simulink model "ClosedLoopStim_SimulatedInput_WithDecoderModel"  (R2016b)
settings: Solver=FixedStepDiscrete  StartTime=0.0  StopTime=inf  FixedStep=sCoreParams.core.stepPeriod  RelTol=1e-3  EnableMultiTasking=on
undefined symbols (not defined in the file or in its folder): sCoreParams, sCoreParams_Features_Baseline_thresholdAboveValue, sCoreParams_Features_Baseline_thresholdBelowValue
libraries: dspswit3 x4, dspsrcs4 x2, simulink x1
settings Model: DataTypeOverride=Double  MinMaxOverflowLogging=ForceOff  Creator=rzelmann  LastModifiedBy=rzelmann
settings SolverCC: EnableConcurrentExecution=on  ConcurrentTasks=on  AutoInsertRateTranBlk=on  InsertRTBMode=Always
settings DataIOCC: SaveFormat=StructureWithTime  SaveOutput=off  SignalLogging=off  DSMLogging=off  SaveTime=off
settings OptimizationCC: BlockReduction=off  OptimizeBlockIOStorage=off  BufferReuse=off  GlobalBufferReuse=off  ExpressionFolding=off  LocalBlockOutputs=off  LifeSpan=inf
settings DebuggingCC: AllowSymbolicDim=off  SFUnexpectedBacktrackingDiag=warning  SFNoUnconditionalDefaultTransitionDiag=warning  SFExecutionAtInitializationDiag=none
settings HardwareCC: ProdBitPerPointer=32  ProdBitPerSizeT=32  ProdBitPerPtrDiffT=32  ProdLargestAtomicFloat=None  ProdWordSize=32  ProdLongLongMode=on  ProdHWDeviceType=Generic->32-bit x86 compatible
settings RTWCC: SystemTargetFile=slrt.tlc  TemplateMakefile=slrt_default_tmf  Description=Simulink Real-Time  RTWCompilerOptimization=on
settings CodeAppCC: MaxIdLength=63
settings ConfigComp: CovMetricSettings=dw  CovHtmlReporting=on  CovSaveCumulativeToWorkspaceVar=on  CovSaveSingleToWorkspaceVar=on  CovExternalEMLEnable=off

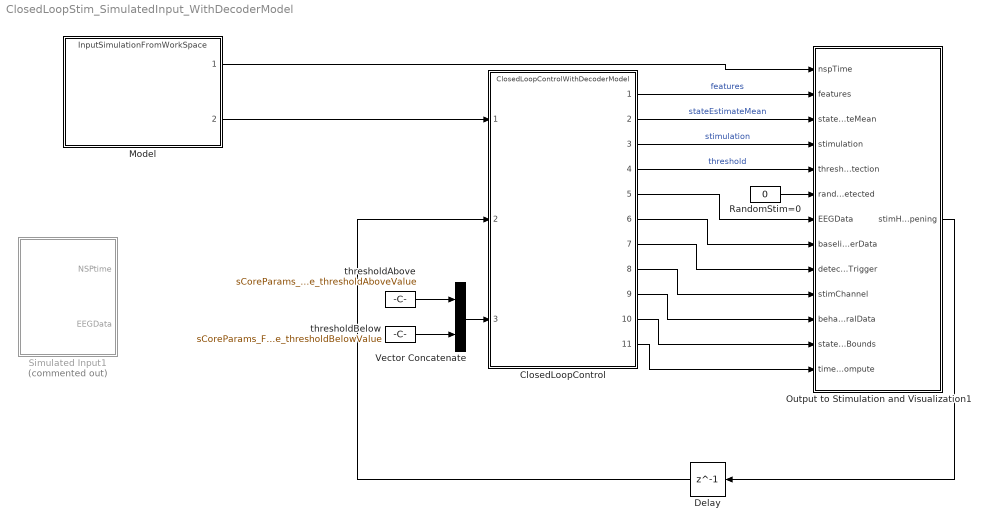
== system ClosedLoopStim_SimulatedInput_WithDecoderModel ==
  ClosedLoopControl : ModelReference  ModelNameDialog=ClosedLoopControlWithDecoderModel.slx  SimulationMode=Normal  ModelReferenceVersion=1.730
  Delay : Delay  DelayLength=1  InitialCondition=0  InputProcessing=Columns as channels (frame based)  SampleTime=sCoreParams.core.stepPeriod
  Model : ModelReference  ModelNameDialog=InputSimulationFromWorkSpace.slx  SimulationMode=Normal  ModelReferenceVersion=1.12
  Output to Stimulation and Visualization1 : Subsystem
  RandomStim=0 : Constant  Value=0  OutDataTypeStr=boolean
  Simulated Input1 : Subsystem  Commented=on
  Vector Concatenate : Concatenate
  thresholdAbove : Constant  Value=sCoreParams_Features_Baseline_thresholdAboveValue
  thresholdBelow : Constant  Value=sCoreParams_Features_Baseline_thresholdBelowValue
  wires:
  Delay/1 -> ClosedLoopControl/2
  ClosedLoopControl/8 -> Output to Stimulation and Visualization1/10(stimChannel)
  ClosedLoopControl/1 -> Output to Stimulation and Visualization1/2(features)  "features"
  ClosedLoopControl/2 -> Output to Stimulation and Visualization1/3(stateEstimateMean)  "stateEstimateMean"
  ClosedLoopControl/3 -> Output to Stimulation and Visualization1/4(stimulation)  "stimulation"
  ClosedLoopControl/4 -> Output to Stimulation and Visualization1/5(thresholdUsedInDetection)  "threshold"
  ClosedLoopControl/6 -> Output to Stimulation and Visualization1/8(baselineTriggerData)
  ClosedLoopControl/7 -> Output to Stimulation and Visualization1/9(detectStimTrigger)
  RandomStim=0/1 -> Output to Stimulation and Visualization1/6(randomDetected)
  ClosedLoopControl/5 -> Output to Stimulation and Visualization1/7(EEGData)
  thresholdAbove/1 -> Vector Concatenate/1
  thresholdBelow/1 -> Vector Concatenate/2
  Vector Concatenate/1 -> ClosedLoopControl/3
  ClosedLoopControl/10 -> Output to Stimulation and Visualization1/12(stateEstimateBounds)
  Output to Stimulation and Visualization1/1(stimHappening) -> Delay/1
  ClosedLoopControl/9 -> Output to Stimulation and Visualization1/11(behavioralData)
  ClosedLoopControl/11 -> Output to Stimulation and Visualization1/13(timeToCompute)
  Model/1 -> Output to Stimulation and Visualization1/1(nspTime)
  Model/2 -> ClosedLoopControl/1

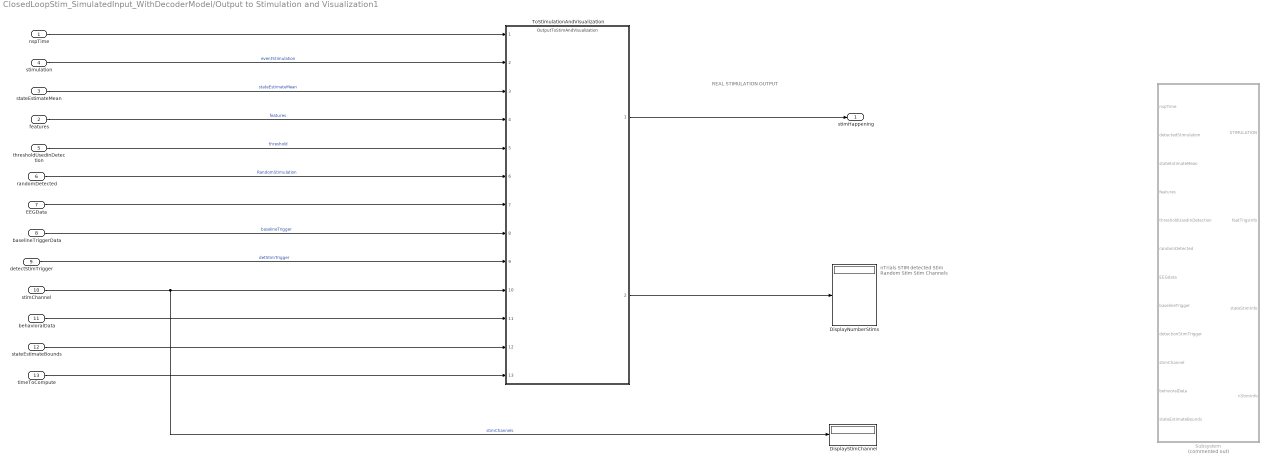
== system ClosedLoopStim_SimulatedInput_WithDecoderModel/Output to Stimulation and Visualization1 ==
  note: nTrials
      | STIM
      | detected Stim
      | Random Stim
      | Stim Channels
  note: REAL STIMULATION OUTPUT
  nspTime : Inport
  features : Inport  Port=2
  stateEstimateMean : Inport  Port=3
  stimulation : Inport  Port=4
  thresholdUsedInDetection : Inport  Port=5
  randomDetected : Inport  Port=6
  EEGData : Inport  Port=7
  baselineTriggerData : Inport  Port=8  OutDataTypeStr=int32
  detectStimTrigger : Inport  Port=9  OutDataTypeStr=int32
  stimChannel : Inport  Port=10
  behavioralData : Inport  Port=11
  stateEstimateBounds : Inport  Port=12
  timeToCompute : Inport  Port=13  OutDataTypeStr=boolean
  DisplayNumberStims : Display
      settings: Format=decimal (Stored Integer)
  DisplayStimChannel : Display
  Subsystem : Subsystem  Commented=on
  ToStimulationAndVisualization : ModelReference  ModelNameDialog=OutputToStimAndVisualization.slx  SimulationMode=Normal  ModelReferenceVersion=1.301
  stimHappening : Outport  OutDataTypeStr=boolean  SampleTime=sCoreParams.core.stepPeriod
  wires:
  stimChannel/1 -> ToStimulationAndVisualization/10, DisplayStimChannel/1  "stimChannels"
  ToStimulationAndVisualization/2 -> DisplayNumberStims/1
  nspTime/1 -> ToStimulationAndVisualization/1
  stimulation/1 -> ToStimulationAndVisualization/2  "eventStimulation"
  stateEstimateMean/1 -> ToStimulationAndVisualization/3  "stateEstimateMean"
  features/1 -> ToStimulationAndVisualization/4  "features"
  thresholdUsedInDetection/1 -> ToStimulationAndVisualization/5  "threshold"
  randomDetected/1 -> ToStimulationAndVisualization/6  "RandomStimulation"
  EEGData/1 -> ToStimulationAndVisualization/7
  baselineTriggerData/1 -> ToStimulationAndVisualization/8  "baselineTrigger"
  detectStimTrigger/1 -> ToStimulationAndVisualization/9  "detStimTrigger"
  behavioralData/1 -> ToStimulationAndVisualization/11
  stateEstimateBounds/1 -> ToStimulationAndVisualization/12
  ToStimulationAndVisualization/1 -> stimHappening/1
  timeToCompute/1 -> ToStimulationAndVisualization/13

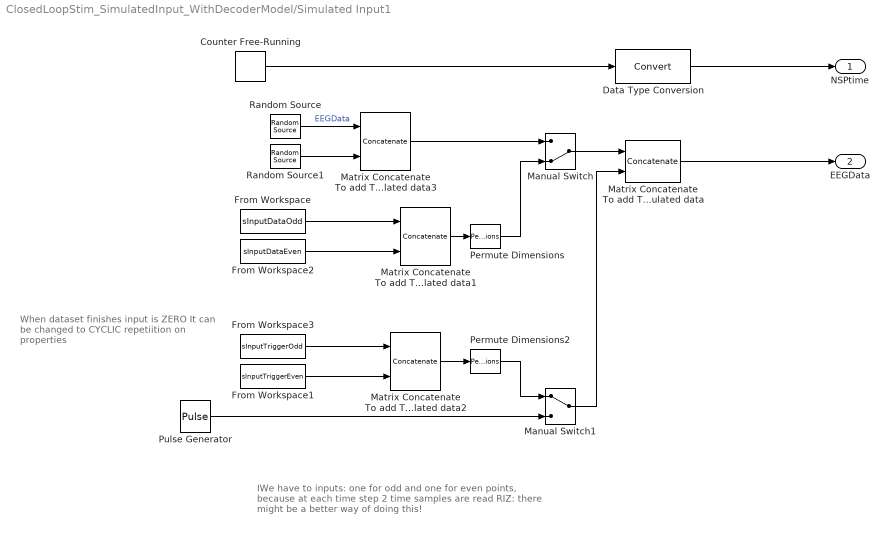
== system ClosedLoopStim_SimulatedInput_WithDecoderModel/Simulated Input1 ==
  note: When dataset finishes input is ZERO
      | It can be changed to CYCLIC repetiition
      | on properties
  note: IWe have to inputs:
      | one for odd and one for even points, because at each time step 2 time samples are read
      | RIZ: there might be a better way of doing this!
  Counter Free-Running : simulink/Sources/Counter Free-Running  NumBits=64  tsamp=sCoreParams.core.stepPeriod
  Data Type Conversion : DataTypeConversion
  From Workspace : FromWorkspace  VariableName=sInputDataOdd  SampleTime=sCoreParams.core.stepPeriod  Interpolate=off  OutputAfterFinalValue=Setting to zero
  From Workspace1 : FromWorkspace  VariableName=sInputTriggerEven  SampleTime=sCoreParams.core.stepPeriod  Interpolate=off  OutputAfterFinalValue=Setting to zero
  From Workspace2 : FromWorkspace  VariableName=sInputDataEven  SampleTime=sCoreParams.core.stepPeriod  Interpolate=off  OutputAfterFinalValue=Setting to zero
  From Workspace3 : FromWorkspace  VariableName=sInputTriggerOdd  SampleTime=sCoreParams.core.stepPeriod  Interpolate=off  OutputAfterFinalValue=Setting to zero
  Manual Switch : ManualSwitch  CurrentSetting=0
  Manual Switch1 : ManualSwitch
  Matrix Concatenate To add Trigger after simulated data : Concatenate  Mode=Multidimensional array  ConcatenateDimension=2
  Matrix Concatenate To add Trigger after simulated data1 : Concatenate  Mode=Multidimensional array  ConcatenateDimension=2
  Matrix Concatenate To add Trigger after simulated data2 : Concatenate  Mode=Multidimensional array  ConcatenateDimension=2
  Matrix Concatenate To add Trigger after simulated data3 : Concatenate  Mode=Multidimensional array
  Permute Dimensions : PermuteDimensions
  Permute Dimensions2 : PermuteDimensions
  Pulse Generator : DiscretePulseGenerator  Amplitude=ones(2,2)  Period=sCoreParams.core.samplingRate * 10  SampleTime=sCoreParams.core.stepPeriod  VectorParams1D=off
  Random Source : dspsrcs4/Random Source  SrcType=Uniform  NormMethod=Ziggurat  CltLength=12  MinVal=-10 * ones(1, sCoreParams.core.maxChannelsAllNSPs-2)  MaxVal=10 * ones(1, sCoreParams.core.maxChannelsAllNSPs-2)  MeanVal=0  VarVal=1  RepMode=Not repeatable  rawSeed=1  IsInherit=off  SampMode=Discrete  SampTime=sCoreParams.core.stepPeriod  SampFrame=1  DataType=Double  OutComplex=Real  OutputFrames=off
  Random Source1 : dspsrcs4/Random Source  SrcType=Uniform  NormMethod=Ziggurat  CltLength=12  MinVal=-10 * ones(1, sCoreParams.core.maxChannelsAllNSPs-2)  MaxVal=10 * ones(1, sCoreParams.core.maxChannelsAllNSPs-2)  MeanVal=0  VarVal=1  RepMode=Not repeatable  rawSeed=1  IsInherit=off  SampMode=Discrete  SampTime=sCoreParams.core.stepPeriod  SampFrame=1  DataType=Double  OutComplex=Real  OutputFrames=off
  NSPtime : Outport
  EEGData : Outport  Port=2
  wires:
  Manual Switch/1 -> Matrix Concatenate To add Trigger after simulated data/1
  Manual Switch1/1 -> Matrix Concatenate To add Trigger after simulated data/2
  Counter Free-Running/1 -> Data Type Conversion/1
  Random Source/1 -> Matrix Concatenate To add Trigger after simulated data3/1  "EEGData"
  Data Type Conversion/1 -> NSPtime/1
  Pulse Generator/1 -> Manual Switch1/2
  Matrix Concatenate To add Trigger after simulated data/1 -> EEGData/1
  Matrix Concatenate To add Trigger after simulated data2/1 -> Permute Dimensions2/1
  From Workspace/1 -> Matrix Concatenate To add Trigger after simulated data1/1
  From Workspace3/1 -> Matrix Concatenate To add Trigger after simulated data2/1
  Matrix Concatenate To add Trigger after simulated data1/1 -> Permute Dimensions/1
  Permute Dimensions/1 -> Manual Switch/2
  Random Source1/1 -> Matrix Concatenate To add Trigger after simulated data3/2
  Matrix Concatenate To add Trigger after simulated data3/1 -> Manual Switch/1
  Permute Dimensions2/1 -> Manual Switch1/1
  From Workspace2/1 -> Matrix Concatenate To add Trigger after simulated data1/2
  From Workspace1/1 -> Matrix Concatenate To add Trigger after simulated data2/2

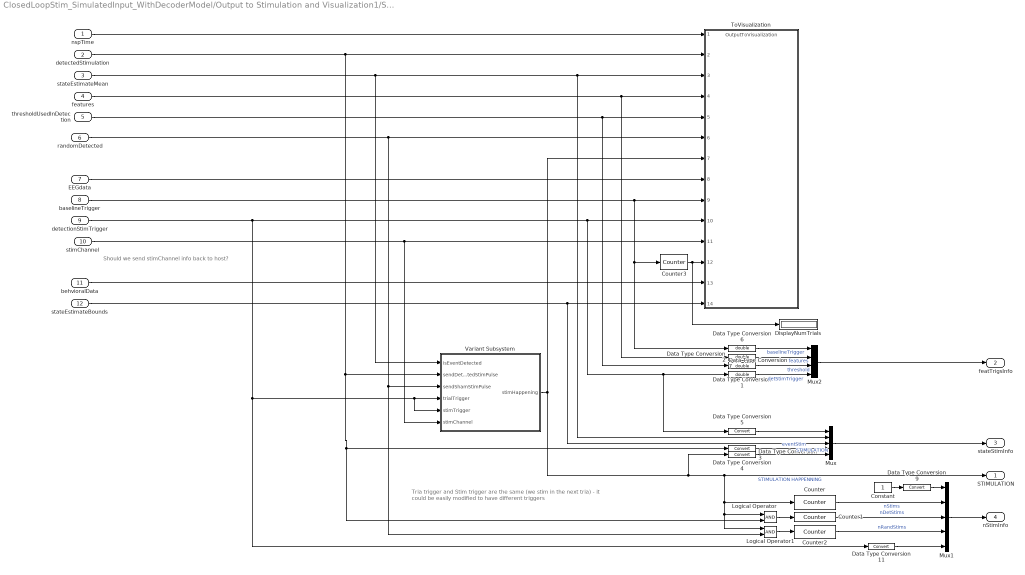
== system ClosedLoopStim_SimulatedInput_WithDecoderModel/Output to Stimulation and Visualization1/Subsystem ==
  note: Should we send stimChannel info back to host?
  note: Tria trigger and Stim trigger are the same (we stim in the next tria)
      | - it could be easily modified to have different triggers
  nspTime : Inport
  detectedStimulation : Inport  Port=2
  stateEstimateMean : Inport  Port=3
  features : Inport  Port=4
  thresholdUsedInDetection : Inport  Port=5
  randomDetected : Inport  Port=6
  EEGdata : Inport  Port=7
  baselineTrigger : Inport  Port=8
  detectionStimTrigger : Inport  Port=9
  stimChannel : Inport  Port=10
  behvioralData : Inport  Port=11
  stateEstimateBounds : Inport  Port=12
  Constant : Constant  OutDataTypeStr=int32
  Counter : dspswit3/Counter  Direction=Up  CountEvent=Rising edge  CounterSize=User defined  MaxCount=1024  InitialCount=0  Output=Count  HitValue=32  ResetInput=off  SamplesPerFrame=1  Ts=1  CntDtype=int32  HitDtype=Logical
  Counter1 : dspswit3/Counter  Direction=Up  CountEvent=Rising edge  CounterSize=User defined  MaxCount=1024  InitialCount=0  Output=Count  HitValue=32  ResetInput=off  SamplesPerFrame=1  Ts=1  CntDtype=int32  HitDtype=Logical
  Counter2 : dspswit3/Counter  Direction=Up  CountEvent=Rising edge  CounterSize=User defined  MaxCount=1024  InitialCount=0  Output=Count  HitValue=32  ResetInput=off  SamplesPerFrame=1  Ts=1  CntDtype=int32  HitDtype=Logical
  Counter3 : dspswit3/Counter  Direction=Up  CountEvent=Rising edge  CounterSize=User defined  MaxCount=1024  InitialCount=0  Output=Count  HitValue=32  ResetInput=off  SamplesPerFrame=1  Ts=1  CntDtype=double  HitDtype=Logical
  Data Type Conversion{1..2,6..7} (4 alike) : DataTypeConversion  OutDataTypeStr=double
  Data Type Conversion{3..5,9,11} (5 alike) : DataTypeConversion
  DisplayNumTrials : Display
  Logical Operator : Logic  IconShape=distinctive  AllPortsSameDT=off  OutDataTypeStr=boolean
  Logical Operator1 : Logic  IconShape=distinctive  AllPortsSameDT=off  OutDataTypeStr=boolean
  Mux : Mux  Inputs=5
  Mux1 : Mux  Inputs=5
  Mux2 : Mux
  ToVisualization : ModelReference  ModelNameDialog=OutputToVisualization  SimulationMode=Normal  ModelReferenceVersion=1.265
  Variant Subsystem : Subsystem  Variant=on
  STIMULATION : Outport
  featTrigsInfo : Outport  Port=2
  stateStimInfo : Outport  Port=3
  nStimInfo : Outport  Port=4
  wires:
  Counter1/1 -> Mux1/3  "nDetStims"
  nspTime/1 -> ToVisualization/1
  Data Type Conversion5/1 -> Mux/1
  behvioralData/1 -> ToVisualization/13
  Data Type Conversion11/1 -> Mux1/5
  detectedStimulation/1 -> Logical Operator/2, Data Type Conversion4/1, Variant Subsystem/2(sendDetectedStimPulse), ToVisualization/2
  Variant Subsystem/1(stimHappening) -> ToVisualization/7, Data Type Conversion3/1, STIMULATION/1, Logical Operator1/1, Logical Operator/1, Counter/1  "STIMULATION HAPPENNING"
  Logical Operator1/1 -> Counter2/1
  detectionStimTrigger/1 -> Data Type Conversion11/1, Variant Subsystem/5(stimTrigger), Variant Subsystem/4(trialTrigger), Data Type Conversion5/1, Data Type Conversion7/1, ToVisualization/10
  Counter3/1 -> DisplayNumTrials/1, ToVisualization/12
  Data Type Conversion6/1 -> Mux2/1  "baselineTrigger"
  Mux2/1 -> featTrigsInfo/1
  Data Type Conversion1/1 -> Mux2/3  "threshold"
  stimChannel/1 -> Variant Subsystem/6(stimChannel), ToVisualization/11
  baselineTrigger/1 -> Data Type Conversion6/1, Counter3/1, ToVisualization/9
  Logical Operator/1 -> Counter1/1
  Data Type Conversion9/1 -> Mux1/1
  stateEstimateMean/1 -> Variant Subsystem/1(isEventDetected), ToVisualization/3, Mux/2
  Counter/1 -> Mux1/2  "nStims"
  Data Type Conversion2/1 -> Mux2/2  "features"
  thresholdUsedInDetection/1 -> Data Type Conversion1/1, ToVisualization/5
  Data Type Conversion4/1 -> Mux/4  "eventStim"
  Mux1/1 -> nStimInfo/1
  Data Type Conversion7/1 -> Mux2/4  "detStimTrigger"
  Constant/1 -> Data Type Conversion9/1
  EEGdata/1 -> ToVisualization/8
  Counter2/1 -> Mux1/4  "nRandStims"
  Data Type Conversion3/1 -> Mux/5  "STIMULATION"
  features/1 -> Data Type Conversion2/1, ToVisualization/4
  Mux/1 -> stateStimInfo/1
  randomDetected/1 -> Logical Operator1/2, Variant Subsystem/3(sendShamStimPulse), ToVisualization/6
  stateEstimateBounds/1 -> Mux/3, ToVisualization/14

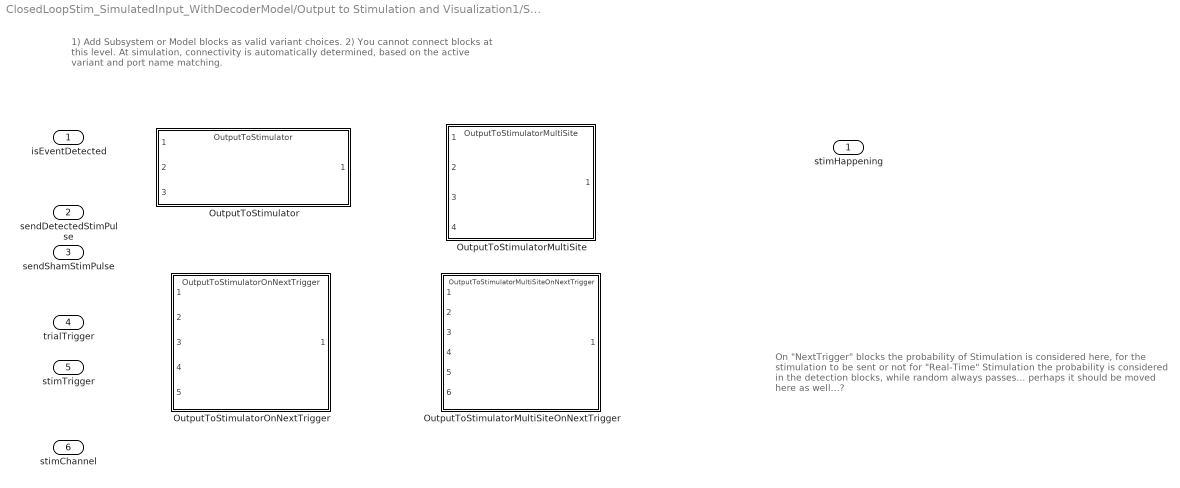
== system ClosedLoopStim_SimulatedInput_WithDecoderModel/Output to Stimulation and Visualization1/Subsystem/Variant Subsystem ==
  note: On "NextTrigger" blocks the probability of Stimulation is considered here,
      | for the stimulation to be sent or not
      | for "Real-Time" Stimulation the probability is considered in the detection blocks,
      | while random always passes... perhaps it should be moved here as well...?
  note: 1) Add Subsystem or Model blocks as valid variant choices.
      | 2) You cannot connect blocks at this level. At simulation, connectivity is automatically
      | determined, based on the active variant and port name matching.
  isEventDetected : Inport
  sendDetectedStimPulse : Inport  Port=2
  sendShamStimPulse : Inport  Port=3
  trialTrigger : Inport  Port=4
  stimTrigger : Inport  Port=5
  stimChannel : Inport  Port=6  OutDataTypeStr=int32
  OutputToStimulator : ModelReference  ModelNameDialog=OutputToStimulator  SimulationMode=Normal  VariantControl=variantParams_STIMULATION_REALTIME  ModelReferenceVersion=1.34
  OutputToStimulatorMultiSite : ModelReference  ModelNameDialog=OutputToStimulatorMultiSite.slx  SimulationMode=Normal  VariantControl=variantParams_STIMULATION_MULTISITE_REALTIME  ModelReferenceVersion=1.48
  OutputToStimulatorMultiSiteOnNextTrigger : ModelReference  ModelNameDialog=OutputToStimulatorMultiSiteOnNextTrigger.slx  SimulationMode=Normal  VariantControl=variantParams_STIMULATION_MULTISITE_NEXTTRIGGER  ModelReferenceVersion=1.85
  OutputToStimulatorOnNextTrigger : ModelReference  ModelNameDialog=OutputToStimulatorOnNextTrigger  SimulationMode=Normal  VariantControl=variantParams_STIMULATION_ONNEXTTRIGGER  ModelReferenceVersion=1.88
  stimHappening : Outport
